simulink model "powerwindow"  (R2017b)
settings: Solver=ode45  StartTime=0.0  StopTime=inf  RelTol=1e-3  EnableMultiTasking=on
settings Model: Creator=ia3803  LastModifiedBy=flosch
settings DataIOCC: LimitDataPoints=on  SaveFormat=Array  SignalLoggingSaveFormat=ModelDataLogs
settings OptimizationCC: ExpressionDepthLimit=2147483647  LifeSpan=inf
settings DebuggingCC: UnderspecifiedInitializationDetection=Classic  MergeDetectMultiDrivingBlocksExec=none  SolverPrmCheckMsg=warning  FcnCallInpInsideContextMsg=warning  StateNameClashWarn=warning  SFUnexpectedBacktrackingDiag=warning  SFNoUnconditionalDefaultTransitionDiag=warning  SFExecutionAtInitializationDiag=none
settings HardwareCC: ProdBitPerPointer=32  ProdBitPerSizeT=32  ProdBitPerPtrDiffT=32  ProdLargestAtomicFloat=None  ProdIntDivRoundTo=Undefined  ProdEndianess=Unspecified  ProdWordSize=32  ProdHWDeviceType=32-bit Generic
settings ModelReferenceCC: PropagateSignalLabelsOutOfModel=off
settings CodeAppCC: StateflowObjectComments=on
settings GRTTargetCC: TargetLangStandard=C89/C90 (ANSI)  GeneratePreprocessorConditionals=Disable all
settings ConfigComp: CovMetricSettings=dw  CovHtmlReporting=on  CovSaveCumulativeToWorkspaceVar=on  CovSaveSingleToWorkspaceVar=on  CovExternalEMLEnable=off

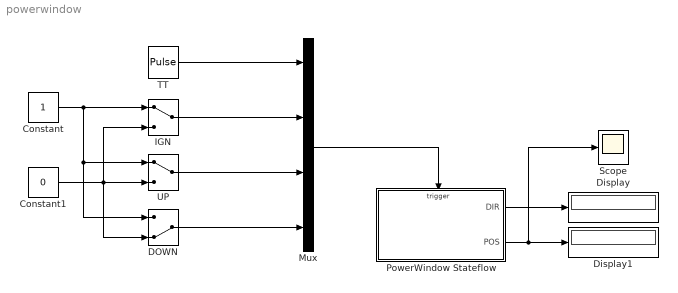
== system powerwindow ==
  Constant : Constant
  Constant1 : Constant  Value=0
  DOWN : ManualSwitch  CurrentSetting=0
  Display : Display
  Display1 : Display
  IGN : ManualSwitch
  Mux : Mux
  PowerWindow Stateflow : Stateflow chart  TreatAsAtomicUnit=on
  Scope : Scope
  TT : DiscretePulseGenerator  PulseType=Time based  Period=1  PulseWidth=50
  UP : ManualSwitch
  wires:
  TT/1 -> Mux/1
  Constant/1 -> IGN/1, UP/1, DOWN/1
  Constant1/1 -> UP/2, DOWN/2, IGN/2
  IGN/1 -> Mux/2
  UP/1 -> Mux/3
  DOWN/1 -> Mux/4
  Mux/1 -> PowerWindow Stateflow/Trigger
  PowerWindow Stateflow/1(DIR) -> Display/1
  PowerWindow Stateflow/2(POS) -> Display1/1, Scope/1

== stateflow chart powerwindow/PowerWindow Stateflow ==
  state ON
    state STANDSTILL
      entry:
      DIR=0;
    state DOWN
      entry:
      DIR=1;
    state UP
      entry:
      DIR=2;
    (default) -> STANDSTILL
    DOWN -> STANDSTILL [order 1] : [POS==0]
    UP -> STANDSTILL [order 2] : [POS==20]
    STANDSTILL -> DOWN [order 1] : DOWN[POS>0]
    STANDSTILL -> UP [order 2] : UP[POS<20]
    UP -> STANDSTILL [order 1] : UP
    DOWN -> STANDSTILL [order 2] : DOWN
    UP -> DOWN [order 4] : DOWN
    DOWN -> UP [order 4] : UP
    DOWN -> DOWN [order 3] : TT[POS>0]/POS--;
    UP -> UP [order 3] : TT[POS<20]/POS++;
  state OFF
  (default) -> OFF : /DIR=0;POS=0;
  OFF -> ON : IGN
  ON -> OFF : IGN
  data: DIR output double; POS output double
  events: TT input EITHER_EDGE_EVENT; IGN input EITHER_EDGE_EVENT; UP input EITHER_EDGE_EVENT; DOWN input EITHER_EDGE_EVENT
